simulink model "sim_Exp81_part5"  (R2019b)
settings: Solver=VariableStepAuto  StartTime=0.0  StopTime=10.0  RelTol=1e-3
undefined symbols (not defined in the file): GP_den, GP_num, Kp_part1, L, T
settings Model: Creator=sgxgong4  LastModifiedBy=xg
settings SFSimCC: CustomCodeUndefinedFunction=UseInterfaceOnly

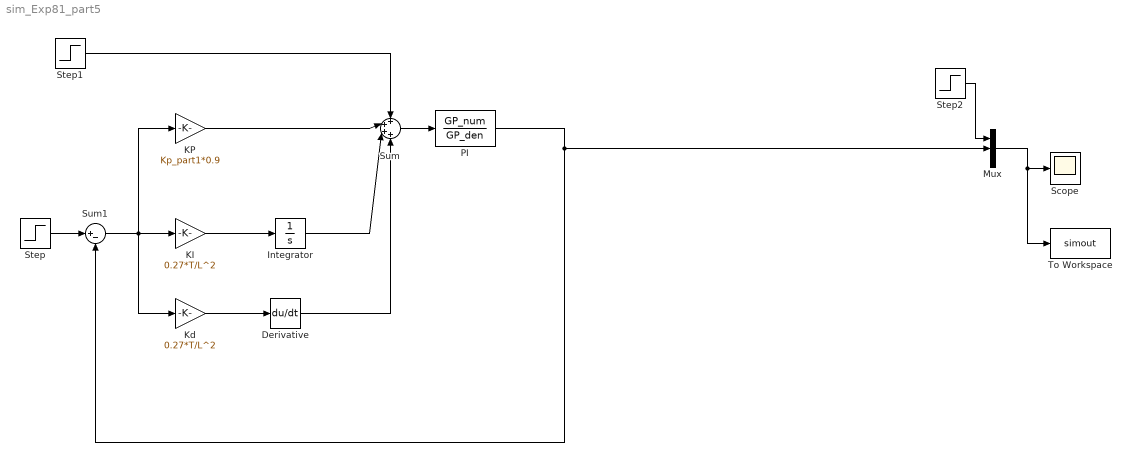
== system sim_Exp81_part5 ==
  Derivative : Derivative
  Integrator : Integrator
  KI : Gain  Gain=0.27*T/L^2
  KP : Gain  Gain=Kp_part1*0.9
  Kd : Gain  Gain=0.27*T/L^2
  Mux : Mux  Inputs=3
  PI : TransferFcn  Numerator=GP_num  Denominator=GP_den
  Scope : Scope
  Step : Step  Time=0  SampleTime=0
  Step1 : Step  Time=0  After=10  SampleTime=0
  Step2 : Step  Time=0  SampleTime=0
  Sum : Sum  Inputs=++++
  Sum1 : Sum  Inputs=|+-
  To Workspace : ToWorkspace  VariableName=simout  SaveFormat=Structure With Time  SampleTime=-1
  wires:
  KI/1 -> Integrator/1
  KP/1 -> Sum/2
  Integrator/1 -> Sum/3
  Step/1 -> Sum1/1
  Sum/1 -> PI/1
  PI/1 -> Sum1/2, Mux/2
  Step1/1 -> Sum/1
  Step2/1 -> Mux/1
  Mux/1 -> To Workspace/1, Scope/1
  Kd/1 -> Derivative/1
  Sum1/1 -> Kd/1, KP/1, KI/1
  Derivative/1 -> Sum/4
